simulink model "sys1"  (R2023b)
settings: Solver=VariableStepAuto  StartTime=0.0  StopTime=30  RelTol=1e-3
settings Model: Creator=xjtu  LastModifiedBy=xjtu

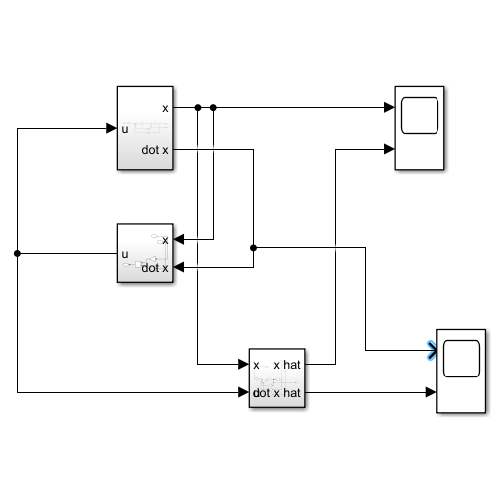
[thumbnail: Simulink's stored preview of the top-level diagram]
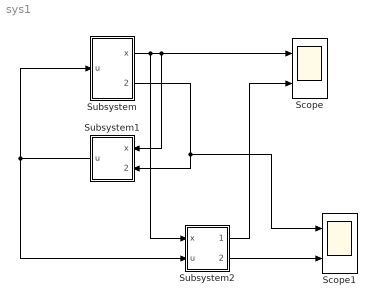
== system sys1 ==
  Scope : Scope  NumInputPorts=2
  Scope1 : Scope  NumInputPorts=2
  Subsystem : Subsystem
  Subsystem1 : Subsystem
  Subsystem2 : Subsystem
  wires:
  Subsystem/2(dot x) -> Scope1/1, Subsystem1/2(dot x)
  Subsystem/1(x) -> Scope/1, Subsystem1/1(x), Subsystem2/1(x)
  Subsystem1/1(u) -> Subsystem/1(u), Subsystem2/2(u)
  Subsystem2/1(x hat) -> Scope/2
  Subsystem2/2(dot x hat) -> Scope1/2

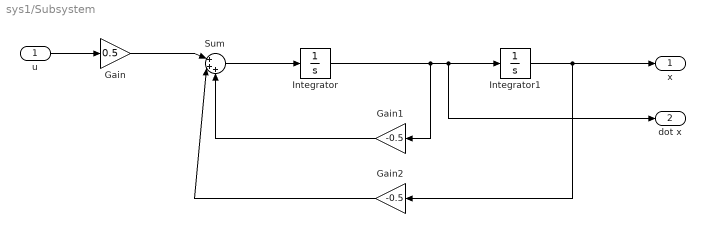
== system sys1/Subsystem ==
  u : Inport
  Gain : Gain  Gain=0.5
  Gain1 : Gain  Gain=-0.5
  Gain2 : Gain  Gain=-0.5
  Integrator : Integrator  InitialCondition=0.2
  Integrator1 : Integrator  InitialCondition=0.5
  Sum : Sum  Inputs=|+++
  x : Outport
  dot x : Outport  Port=2
  wires:
  Integrator1/1 -> x/1, Gain2/1
  Sum/1 -> Integrator/1
  Gain1/1 -> Sum/3
  Integrator/1 -> Gain1/1, dot x/1, Integrator1/1
  Gain2/1 -> Sum/2
  u/1 -> Gain/1
  Gain/1 -> Sum/1

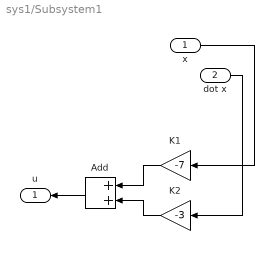
== system sys1/Subsystem1 ==
  x : Inport
  dot x : Inport  Port=2
  Add : Sum
  K1 : Gain  Gain=-7
  K2 : Gain  Gain=-3
  u : Outport
  wires:
  dot x/1 -> K2/1
  K1/1 -> Add/1
  K2/1 -> Add/2
  x/1 -> K1/1
  Add/1 -> u/1

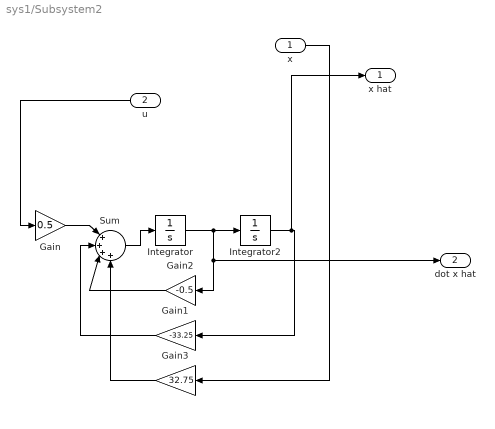
== system sys1/Subsystem2 ==
  x : Inport
  u : Inport  Port=2
  Gain : Gain  Gain=0.5
  Gain1 : Gain  Gain=-33.25
  Gain2 : Gain  Gain=-0.5
  Gain3 : Gain  Gain=32.75
  Integrator : Integrator
  Integrator2 : Integrator  InitialCondition=0.5
  Sum : Sum  Inputs=|++++
  x hat : Outport
  dot x hat : Outport  Port=2
  wires:
  Gain1/1 -> Sum/2
  Gain2/1 -> Sum/3
  Gain3/1 -> Sum/4
  Integrator/1 -> dot x hat/1, Gain2/1, Integrator2/1
  x/1 -> Gain3/1
  Integrator2/1 -> x hat/1, Gain1/1
  Gain/1 -> Sum/1
  Sum/1 -> Integrator/1
  u/1 -> Gain/1
